simulink model "Simulink_System1"  (R2020a)
settings: Solver=VariableStepAuto  StartTime=0.0  StopTime=10.0  MaxStep=0.001  RelTol=1e-3
undefined symbols (not defined in the file): a, k1, kcA1, kdA1, kiA1
libraries: cstblocks x3, simulink x1
settings Model: Creator=beto1  LastModifiedBy=beto1

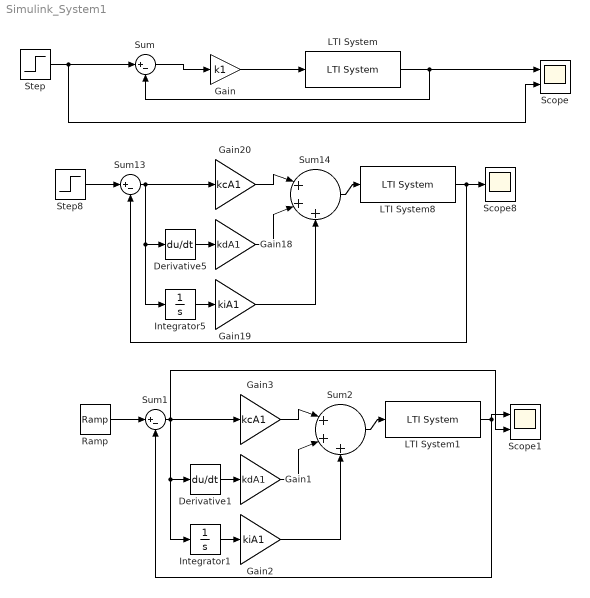
== system Simulink_System1 ==
  Derivative1 : Derivative
  Derivative5 : Derivative
  Gain : Gain  Gain=k1
  Gain1 : Gain  Gain=kdA1
  Gain18 : Gain  Gain=kdA1
  Gain19 : Gain  Gain=kiA1
  Gain2 : Gain  Gain=kiA1
  Gain20 : Gain  Gain=kcA1
  Gain3 : Gain  Gain=kcA1
  Integrator1 : Integrator
  Integrator5 : Integrator
  LTI System : cstblocks/LTI System  sys=G1  IC=[]
  LTI System1 : cstblocks/LTI System  sys=G1  IC=[]
  LTI System8 : cstblocks/LTI System  sys=G1  IC=[]
  Ramp : simulink/Sources/Ramp  slope=a  start=0  InitialOutput=0
  Scope : Scope  NumInputPorts=2
  Scope1 : Scope  NumInputPorts=2
  Scope8 : Scope
  Step : Step  Time=0  SampleTime=0
  Step8 : Step  Time=0  After=8  SampleTime=0
  Sum : Sum  Inputs=|+-
  Sum1 : Sum  Inputs=|+-
  Sum13 : Sum  Inputs=|+-
  Sum14 : Sum  Inputs=|+++
  Sum2 : Sum  Inputs=|+++
  wires:
  Gain/1 -> LTI System/1
  Sum/1 -> Gain/1
  Step/1 -> Sum/1, Scope/2
  LTI System/1 -> Sum/2, Scope/1
  Gain19/1 -> Sum14/3
  Gain20/1 -> Sum14/1
  Sum14/1 -> LTI System8/1
  Gain18/1 -> Sum14/2
  Step8/1 -> Sum13/1
  Derivative5/1 -> Gain18/1
  LTI System8/1 -> Sum13/2, Scope8/1
  Integrator5/1 -> Gain19/1
  Sum13/1 -> Integrator5/1, Derivative5/1, Gain20/1
  Integrator1/1 -> Gain2/1
  Sum1/1 -> Scope1/2, Integrator1/1, Derivative1/1, Gain3/1
  LTI System1/1 -> Sum1/2, Scope1/1
  Gain2/1 -> Sum2/3
  Sum2/1 -> LTI System1/1
  Gain3/1 -> Sum2/1
  Derivative1/1 -> Gain1/1
  Gain1/1 -> Sum2/2
  Ramp/1 -> Sum1/1
